simulink model "Missile_simulink_model"  (R2019b)
settings: Solver=VariableStepAuto  StartTime=0.0  StopTime=80  RelTol=1e-3
values from neighbouring files (symbols this model uses):
  A = [-1.064 1.000; 290.26 0.00]    [Missile_param_1.m]
  B = [-0.25; -331.40]    [Missile_param_1.m]
  C = [-123.34 0.00; 0.00 1.00]    [Missile_param_1.m]
  D = [-13.51; 0]    [Missile_param_1.m]
  dT1 = 0.75    [Missile_param_1.m]
  dT2 = 0.25    [Missile_param_1.m]
  ELEV_INIT = 10000    [Missile_param_1.m]
  ELEV_OBS = 6500    [Missile_param_1.m]    (also in fcn.m = OBS(3))
  ELEV_TARGET = 795    [Missile_param_1.m]    (also in fcn.m = TARGET(3))
  LAT_INIT = 34.2329    [Missile_param_1.m]
  LAT_OBS = 34.453739    [Missile_param_1.m]    (also in fcn.m = OBS(1))
  LAT_TARGET = 34.6588    [Missile_param_1.m]    (also in fcn.m = TARGET(1))
  LON_INIT = -119.4573    [Missile_param_1.m]
  LON_OBS = -119.097053    [Missile_param_1.m]    (also in fcn.m = OBS(2))
  LON_TARGET = -118.769745    [Missile_param_1.m]    (also in fcn.m = TARGET(2))
  Vel = 1021.08    [Missile_param_1.m]
undefined symbols (not defined in the file or in its folder): Earth, K, L, WGS84
libraries: simulink x4, aerolibtransform2 x1, aerolibanimutils x1
settings Model: Creator=USER  LastModifiedBy=USER

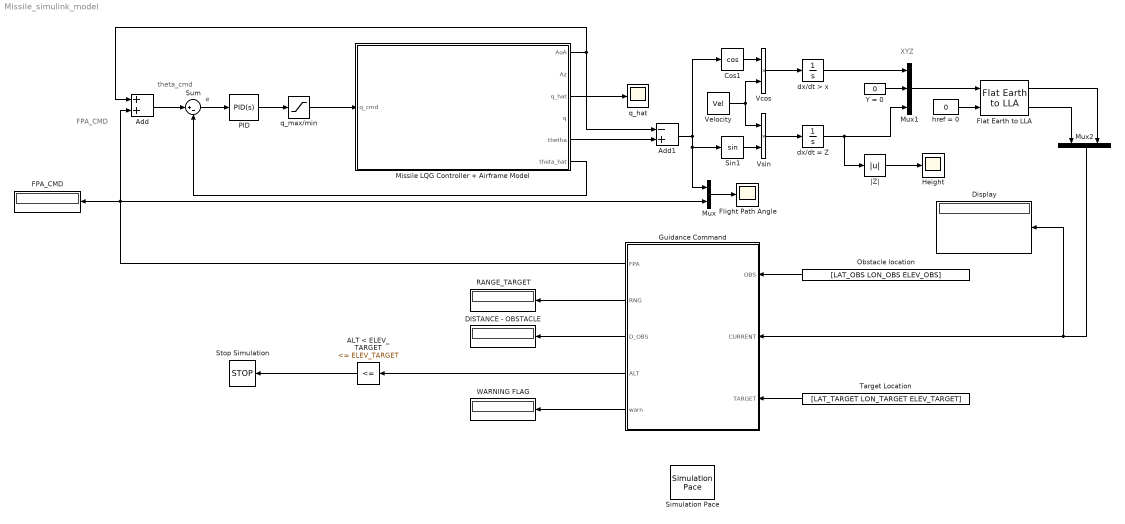
== system Missile_simulink_model ==
  note: XYZ
  note: FPA_CMD
  note: theta_cmd
  note: e
  ALT < ELEV_TARGET : simulink/Logic and Bit Operations/Compare To Constant  relop=<=  const=ELEV_TARGET  OutDataTypeStr=boolean
  Add : Sum
  Add1 : Sum  Inputs=-+
  Cos1 : Trigonometry  Operator=cos
  DISTANCE - OBSTACLE : Display
  Display : Display
  FPA_CMD : Display
  Flat Earth to LLA : aerolibtransform2/Flat Earth to LLA  units=Metric (MKS)  ptype=Earth (WGS84)  F=1/298.257223563  R=6378137  LL0=[LAT_INIT LON_INIT]  psi=yaw_init
  Flight Path Angle : Scope
  Guidance Command : MATLAB Function  TreatAsAtomicUnit=on
  Height : Scope
  Missile LQG Controller + Airframe Model : Subsystem
  Mux : Mux  Inputs=2
  Mux1 : Mux  Inputs=3
  Mux2 : Mux  Inputs=2
  Obstacle location : Constant  Value=[LAT_OBS LON_OBS ELEV_OBS]  VectorParams1D=off
  "PID " : simulink/Continuous/PID Controller  Controller=PID  Form=Parallel  TimeDomain=Continuous-time  SampleTime=-1  IntegratorMethod=Forward Euler  FilterMethod=Forward Euler  ControllerParametersSource=internal  P=-1  I=0  D=0  UseFilter=on  N=100  TunerSelectOption=Transfer Function Based (PID Tuner App)  InitialConditionSource=internal  InitialConditionForIntegrator=0  InitialConditionForFilter=0  DifferentiatorICPrevScaledInput=0  ExternalReset=none  TrackingMode=off  Kt=1  LimitOutput=off  UpperSaturationLimit=inf  LowerSaturationLimit=-inf  LinearizeAsGain=on  AntiWindupMode=none  Kb=1  POutMin=[]  POutMax=[]  IOutMin=[]  IOutMax=[]  DOutMin=[]  DOutMax=[]  NOutMin=[]  NOutMax=[]  SumOutMin=[]  SumOutMax=[]  SaturationOutMin=[]  SaturationOutMax=[]  PParamMin=[]  PParamMax=[]  IParamMin=[]  IParamMax=[]  DParamMin=[]  DParamMax=[]  NParamMin=[]  NParamMax=[]  KbParamMin=[]  KbParamMax=[]  KtParamMin=[]  KtParamMax=[]  KbOutMin=[]  KbOutMax=[]  KtOutMin=[]  KtOutMax=[]  IntegratorOutMin=[]  IntegratorOutMax=[]  FilterOutMin=[]  FilterOutMax=[]  SumI1OutMin=[]  SumI1OutMax=[]  SumI2OutMin=[]  SumI2OutMax=[]  SumI3OutMin=[]  SumI3OutMax=[]  SumI4OutMin=[]  SumI4OutMax=[]  SumDOutMin=[]  SumDOutMax=[]  DifferentiatorOutMin=[]  DifferentiatorOutMax=[]  FilterDiffOutCoefMin=[]  FilterDiffOutCoefMax=[]  ReciprocalOutMin=[]  ReciprocalOutMax=[]  SumDenOutMin=[]  SumDenOutMax=[]  SumNumOutMin=[]  SumNumOutMax=[]  DivideOutMin=[]  DivideOutMax=[]  IntegratorContinuousStateAttributes=''  IntegratorStateMustResolveToSignalObject=off  IntegratorRTWStateStorageClass=Auto  FilterContinuousStateAttributes=''  FilterStateMustResolveToSignalObject=off  FilterRTWStateStorageClass=Auto  ParallelPVariant=InternalParameters  IdealPVariant=Disabled  IVariant=InternalParameters  DVariant=InternalParameters  IntegratorVariant=Continuous  SatVariant=Disabled  AWVariant=Passthrough  PCopyVariant=Disabled  TRVariant=Disabled  FdbkBlocksVariant=Forward  IdealPFdbkVariant=Disabled  SatFdbkVariant=Disabled  DerivativeFilterVariant=ContFilter  NVariant=InternalParameters  NCopyVariant=Disabled  FilterICVariant=InternalICsFilter  IntegratorICVariant=InternalICs  ExternalResetVariant=Disabled  TRSumVariant=Passthrough  SumFdbkVariant=Disabled  SumVariant=Sum_PID
  RANGE_TARGET : Display
  Simulation Pace : aerolibanimutils/Simulation Pace  SimulationPace=2  SleepMode=MATLAB Thread  OutputPaceError=off  SampleTime=1/30
  Sin1 : Trigonometry
  Stop Simulation : Stop
  Sum : Sum  Inputs=|+-
  Target Location : Constant  Value=[LAT_TARGET LON_TARGET ELEV_TARGET]  VectorParams1D=off
  Vcos : Product
  Velocity : Constant  Value=Vel
  Vsin : Product
  WARNING FLAG : Display
  Y = 0 : Constant  Value=0
  dx/dt = Z : Integrator  InitialCondition=-ELEV_INIT
  dx/dt > x : Integrator
  href = 0 : Constant  Value=0
  q_hat : Scope
  q_max/min : Saturate
  |Z| : Abs
  wires:
  q_max/min/1 -> Missile LQG Controller + Airframe Model/1("q_cmd ")
  "PID "/1 -> q_max/min/1
  Missile LQG Controller + Airframe Model/6(theta_hat) -> Sum/2
  Sum/1 -> "PID "/1
  Add/1 -> Sum/1
  Missile LQG Controller + Airframe Model/1(AoA) -> Add/1, Add1/1
  Missile LQG Controller + Airframe Model/5(thetha) -> Add1/2
  Add1/1 -> Cos1/1, Sin1/1, Mux/1
  Mux/1 -> Flight Path Angle/1
  Sin1/1 -> Vsin/2
  Cos1/1 -> Vcos/1
  Velocity/1 -> Vsin/1, Vcos/2
  Vcos/1 -> dx/dt > x/1
  Vsin/1 -> dx/dt = Z/1
  dx/dt > x/1 -> Mux1/1
  Y = 0/1 -> Mux1/2
  dx/dt = Z/1 -> |Z|/1, Mux1/3
  |Z|/1 -> Height/1
  Mux1/1 -> Flat Earth to LLA/1
  href = 0/1 -> Flat Earth to LLA/2
  Flat Earth to LLA/2 -> Mux2/1
  Flat Earth to LLA/1 -> Mux2/2
  Obstacle location/1 -> Guidance Command/1(OBS)
  Target Location/1 -> Guidance Command/3(TARGET)
  Mux2/1 -> Display/1, Guidance Command/2(CURRENT)
  Guidance Command/2(RNG) -> RANGE_TARGET/1
  Guidance Command/3(D_OBS) -> DISTANCE - OBSTACLE/1
  Guidance Command/5(warn) -> WARNING FLAG/1
  Guidance Command/1(FPA) -> Add/2, FPA_CMD/1, Mux/2
  Guidance Command/4(ALT) -> ALT < ELEV_TARGET/1
  ALT < ELEV_TARGET/1 -> Stop Simulation/1
  Missile LQG Controller + Airframe Model/3(q_hat) -> q_hat/1

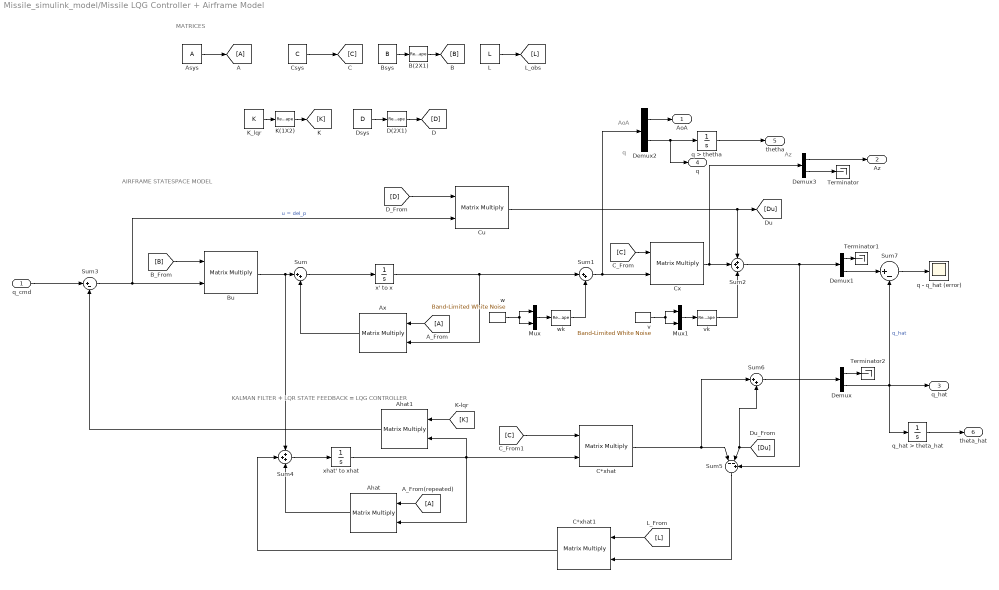
== system Missile_simulink_model/Missile LQG Controller + Airframe Model ==
  note: Az
  note: q
  note: AoA
  note: AIRFRAME STATESPACE MODEL
  note: KALMAN FILTER + LQR STATE FEEDBACK = LQG CONTROLLER
  note: MATRICES
  "q_cmd " : Inport
  Ahat : Product  Multiplication=Matrix(*)
  Ahat1 : Product  Multiplication=Matrix(*)
  Asys : Constant  Value=A
  Ax : Product  Multiplication=Matrix(*)
  B(2X1) : Reshape  OutputDimensionality=Customize  OutputDimensions=[2,1]
  Bsys : Constant  Value=B
  Bu : Product  Multiplication=Matrix(*)
  C*xhat : Product  Multiplication=Matrix(*)
  C*xhat1 : Product  Multiplication=Matrix(*)
  Csys : Constant  Value=C
  Cu : Product  Multiplication=Matrix(*)
  Cx : Product  Multiplication=Matrix(*)
  D(2X1) : Reshape  OutputDimensionality=Customize  OutputDimensions=[2,1]
  Demux{,1..3} (4 alike) : Demux  Outputs=2
  Dsys : Constant  Value=D
  K(1X2) : Reshape  OutputDimensionality=Customize  OutputDimensions=[1,2]
  K_lqr : Constant  Value=K
  "L " : Constant  Value=L
  Mux : Mux  Inputs=2
  Mux1 : Mux  Inputs=2
  Sum : Sum  Inputs=|++
  Sum1 : Sum  Inputs=|++
  Sum2 : Sum  Inputs=+++
  Sum3 : Sum  Inputs=|+-
  Sum4 : Sum  Inputs=+++
  Sum5 : Sum  Inputs=|--+
  Sum6 : Sum  Inputs=|++
  Sum7 : Sum  Inputs=|+-
  Terminator : Terminator
  Terminator1 : Terminator
  Terminator2 : Terminator
  q - q_hat (error) : Scope
  q > thetha : Integrator
  q_hat > theta_hat : Integrator
  v : simulink/Sources/Band-Limited White Noise  Cov=[0.00001]  Ts=dT2  seed=[23341]
  vk : Reshape  OutputDimensionality=Customize  OutputDimensions=[2,1]
  w : simulink/Sources/Band-Limited White Noise  Cov=[0.00000001]  Ts=dT1  seed=[23341]
  wk : Reshape  OutputDimensionality=Customize  OutputDimensions=[2,1]
  x' to x : Integrator
  xhat' to xhat : Integrator
  AoA : Outport
  Az : Outport  Port=2
  q_hat : Outport  Port=3
  q : Outport  Port=4
  thetha : Outport  Port=5
  theta_hat : Outport  Port=6
  wires:
  Demux/1 -> Terminator2/1
  "q_cmd "/1 -> Sum3/1
  Cu/1 -> Sum2/1, [Du]
  Cx/1 -> Demux3/1, Sum2/2
  Ahat/1 -> Sum4/3
  Ax/1 -> Sum/2
  Sum3/1 -> Cu/2, Bu/2  "u = del_p"
  xhat' to xhat/1 -> Ahat1/2, C*xhat/2, Ahat/2
  wk/1 -> Sum1/2
  Demux/2 -> q_hat/1, Sum7/2, q_hat > theta_hat/1  "q_hat"
  [A] -> Ax/1
  Sum5/1 -> C*xhat1/2
  v/1 -> Mux1/1, Mux1/2
  Sum2/1 -> Demux1/1, Sum5/3
  Mux/1 -> wk/1
  x' to x/1 -> Ax/2, Sum1/1
  [D] -> Cu/1
  Demux2/2 -> q/1, q > thetha/1
  Sum6/1 -> Demux/1
  [A] -> Ahat/1
  [C] -> C*xhat/1
  w/1 -> Mux/1, Mux/2
  Csys/1 -> [C]
  Bsys/1 -> B(2X1)/1
  Demux2/1 -> AoA/1
  K_lqr/1 -> K(1X2)/1
  C*xhat1/1 -> Sum4/2
  Demux1/1 -> Terminator1/1
  Sum1/1 -> Cx/2, Demux2/1
  Ahat1/1 -> Sum3/2
  Sum4/1 -> xhat' to xhat/1
  [B] -> Bu/1
  "L "/1 -> [L]
  C*xhat/1 -> Sum6/1, Sum5/1
  Bu/1 -> Sum/1, Sum4/1
  [C] -> Cx/1
  D(2X1)/1 -> [D]
  Demux3/2 -> Terminator/1
  B(2X1)/1 -> [B]
  Demux3/1 -> Az/1
  Demux1/2 -> Sum7/1
  [Du] -> Sum6/2, Sum5/2
  Sum7/1 -> q - q_hat (error)/1
  K(1X2)/1 -> [K]
  Dsys/1 -> D(2X1)/1
  q > thetha/1 -> thetha/1
  [K] -> Ahat1/1
  q_hat > theta_hat/1 -> theta_hat/1
  [L] -> C*xhat1/1
  Mux1/1 -> vk/1
  vk/1 -> Sum2/3
  Sum/1 -> x' to x/1
  Asys/1 -> [A]

== matlab function Missile_simulink_model/Guidance Command ==
  data: OBS input; FPA output; CURRENT input; TARGET input; RNG output; D_OBS output; ALT output; warn output
function [FPA, RNG, D_OBS, ALT, warn] = fcn(OBS, CURRENT, TARGET)

d2r = pi / 180;   %degree to radians
R = 6371e3;

% OBSTACLE LOCATION
LAT_OBS = OBS(1);
LON_OBS = OBS(2);
ELEV_OBS = OBS(3);

% OBSTACLE THRESHOLD ZONE
thres = 3000;

% TARGET LOCATION
LAT_TARGET = TARGET(1);
LON_TARGET = TARGET(2);
ELEV_TARGET = TARGET(3);

% CURRENT LOCATION
ELEV_CUR = CURRENT(1);
LAT_CUR = CURRENT(2);
LON_CUR = CURRENT(3);

% DISTANCE TO TARGET
l1 = LAT_CUR*d2r;
u1 = LON_CUR*d2r;
l2 = LAT_TARGET*d2r;
u2 = LON_TARGET*d2r;
dh = abs(ELEV_TARGET - ELEV_CUR);

d1 = l2 - l1;
du = u2 - u1;

%harveersine formula (distance across the floor not the range)
a = sin(d1/2)^2 + cos(l1)*cos(l2)*sin(du/2)^2; 
c = 2*atan2(sqrt(a),sqrt(1-a));
d = R*c; % horizontal distance (in m);

% DISTANCE FROM THE OBSTACLE
l3 = LAT_OBS*d2r;
u3 = LON_OBS*d2r;

d1 = l3 - l1;
du = u3 - u1;

a = sin(d1/2)^2 + cos(l1)*cos(l2)*sin(du/2)^2; 
c = 2*atan2(sqrt(a),sqrt(1-a));
d_obs = R*c; 

% current range (from target) - range > distance
range = sqrt(d^2 + dh^2);

%calculate commanded flight path setpoint based on d_obs, range

% if abs(d_obs) >= thres
%     w = 0;
%     FPA_CMD = atan(dh/d);
% else
%     w = 1;
%     FPA_CMD = 0;
% end
if abs(d_obs) >= thres
    w = 0;
    FPA_CMD = atan(dh/d);
else
    w = 1;
    FPA_CMD = atan(-abs((ELEV_CUR*1.01 - ELEV_OBS)/d_obs));
end
FPA = FPA_CMD;
RNG = range;
D_OBS = d_obs;
ALT = ELEV_CUR;
warn = w;
